simulink model "Simulation"  (R2018a)
settings: Solver=VariableStepAuto  StartTime=0.0  StopTime=10  FixedStep=1e-6  MaxStep=Tsc  RelTol=1e-3  EnableMultiTasking=on
InitFcn:
  | clc
  | close all
  | clear all
  | 
  | %Vector-space-decomposition transform (2)
  | D = 2/6*[cos(0) cos(1*pi/3) cos(2*pi/3) cos(3*pi/3) cos(4*pi/3) cos(5*pi/3);
  |         sin(0) sin(1*pi/3) sin(2*pi/3) sin(3*pi/3) sin(4*pi/3) sin(5*pi/3);
  |         cos(2*0) cos(2*pi/3) cos(4*pi/3) cos(6*pi/3) cos(8*pi/3) cos(10*pi/3);
  |         sin(2*0) sin(2*pi/3) sin(4*pi/3) sin(6*pi/3) sin(8*pi/3) sin(10*pi/3);
  |         1/2 1/2  1/2 1/2 1/2 1/2;
  |         1/2 -1/2 1/2 -1/2 1/2 -1/2];
  | 
  | %Control sampling period
  | Tsc = 1e-4;
  | 
  | %Parameters of six-phase induction machine (other than stator resistance):
  | P=2; %Number of machine pole pairs
  | Lm=284e-3; %alpha-beta magnetizing inductance (mH)
  | Rr=2.9; %alpha-beta rotor resistance (ohm)
  | Lls=10e-3; %alpha-beta stator leakage inductance (mH)
  | Llr=21e-3; %alpha-beta rotor leakage inductance (mH)
  | Lxy=4.52e-3; %xy stator inductance (mH)
  | L0=24.5e-3; %0- stator inductance (mH)
  | J=0.0261; %Inertia (Kg*m^2)
  | f=0.0033; %Friction coefficient (N*m*s)
  | Ls = Lls+Lm; Lr = Llr+Lm;  %alpha-beta self-inductances (mH)
undefined symbols (not defined in the file): DiscIntNeverNeededParam
libraries: powerlib x37, simulink x20, simulink_extras x7
(part 2 of 3)

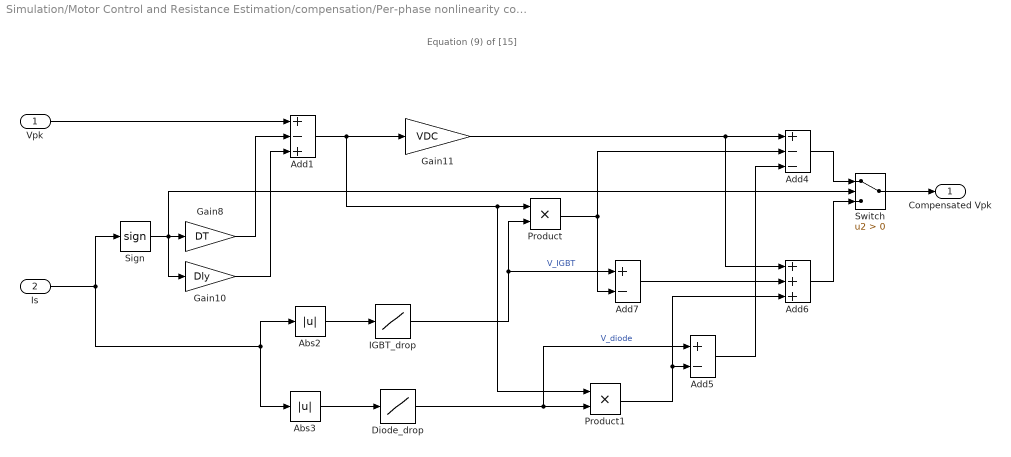
== system Simulation/Motor Control and Resistance Estimation/compensation/Per-phase nonlinearity comp. a ==
  note: Equation (9) of [15]
  Vpk : Inport
  Is : Inport  Port=2
  Abs2 : Abs
  Abs3 : Abs
  Add1 : Sum  Inputs=+-+
  Add4 : Sum  Inputs=+--
  Add5 : Sum  Inputs=+-
  Add6 : Sum  Inputs=+++
  Add7 : Sum  Inputs=+-
  Diode_drop : Lookup_n-D  NumberOfTableDimensions=1  BreakpointsForDimension1=|  Table=|  InternalRulePriority=Speed  RndMeth=Simplest  InputSameDT=on
      BreakpointsForDimension1=|
      | [0
      | 0.133928966
      | 0.255064642
      | 0.474221552
      | 0.729904408
      | 0.949060092
      | 1.31432079
      | 1.606529594
      | 1.935264345
      | 2.337050991
      | 2.665784516
      | 3.031045214
      | 3.286728071
      | 3.688514717
      | 4.090301362
      | 4.528613955
      | 4.966926548
      | 5.369012486
      | 6.011863029
      | 6.494000937
      | 6.895782526
      | 7.538633069
      | 7.940414658
      | 8.392857318
      | 9.017857931
      | 9.508928352
      | 10.04464299
      | 10.53571464
      | 11.07142805
      | 11.60714268
      | 12.09821433
      | ]
      Table=|
      | [0.649155738
      | 0.724202664
      | 0.757646637
      | 0.789882494
      | 0.820583364
      | 0.852819221
      | 0.883520091
      | 0.906545718
      | 0.924966281
      | 0.949526998
      | 0.971017535
      | 0.987903009
      | 1.006323572
      | 1.021673955
      | 1.040094519
      | 1.058514979
      | 1.075400452
      | 1.095506677
      | 1.110703514
      | 1.130965963
      | 1.15291695
      | 1.164736713
      | 1.184999162
      | 1.206378996
      | 1.217636169
      | 1.228893136
      | 1.240150103
      | 1.255159529
      | 1.264540369
      | 1.281425922
      | 1.300187602
      | ]
  Gain10 : Gain  Gain=Dly
  Gain11 : Gain  Gain=VDC
  Gain8 : Gain  Gain=DT
  IGBT_drop : Lookup_n-D  NumberOfTableDimensions=1  BreakpointsForDimension1=|  Table=|  InternalRulePriority=Speed  RndMeth=Simplest  InputSameDT=on
      BreakpointsForDimension1=|
      | [0
      | 0.18153084
      | 0.386589315
      | 0.625825349
      | 0.933414208
      | 1.309355891
      | 1.651121163
      | 2.129592084
      | 2.53971018
      | 3.052357513
      | 3.530829581
      | 3.872593705
      | 4.385242186
      | 4.658654632
      | 5.034596316
      | 5.37636044
      | 5.752302124
      | 6.059890983
      | 6.401656254
      | 6.743421525
      | 7.085186797
      | 7.426952068
      | 7.802893752
      | 8.110482611
      | 8.38389391
      | 8.588953532
      | 8.89654239
      | 9.238307662
      | 9.443366136
      | 9.68260217
      | 9.921837631
      | 10.22942592
      | 10.53701477
      | 10.91295646
      | 11.11801551
      | 11.39142738
      | 11.73319265
      | 12.04078151
      | ]
      Table=|
      | [0.58448405
      | 0.632969591
      | 0.671758056
      | 0.708122171
      | 0.739637748
      | 0.783274751
      | 0.817214515
      | 0.858427331
      | 0.880245832
      | 0.899639983
      | 0.921458485
      | 0.948125524
      | 0.969944025
      | 0.984489639
      | 1.00388379
      | 1.023278104
      | 1.037823717
      | 1.059642218
      | 1.071763644
      | 1.086309258
      | 1.100854871
      | 1.112976297
      | 1.12752191
      | 1.144491874
      | 1.154188949
      | 1.166310375
      | 1.173583101
      | 1.188128877
      | 1.197825952
      | 1.209947378
      | 1.222068641
      | 1.234190067
      | 1.239038605
      | 1.246311493
      | 1.258432919
      | 1.270554182
      | 1.280251257
      | 1.289948496
      | ]
  Product : Product
  Product1 : Product
  Sign : Signum
  Switch : Switch  Criteria=u2 > Threshold
  Compensated Vpk : Outport
  wires:
  Add6/1 -> Switch/3
  Is/1 -> Abs3/1, Abs2/1, Sign/1
  Product1/1 -> Add6/3, Add5/2
  Add1/1 -> Product1/1, Product/1, Gain11/1
  Product/1 -> Add7/2, Add4/2
  Diode_drop/1 -> Add5/1, Product1/2  "V_diode"
  Sign/1 -> Switch/2, Gain10/1, Gain8/1
  Add7/1 -> Add6/2
  Gain11/1 -> Add6/1, Add4/1
  Add4/1 -> Switch/1
  Gain8/1 -> Add1/2
  IGBT_drop/1 -> Add7/1, Product/2  "V_IGBT"
  Add5/1 -> Add4/3
  Abs2/1 -> IGBT_drop/1
  Gain10/1 -> Add1/3
  Switch/1 -> Compensated Vpk/1
  Vpk/1 -> Add1/1
  Abs3/1 -> Diode_drop/1

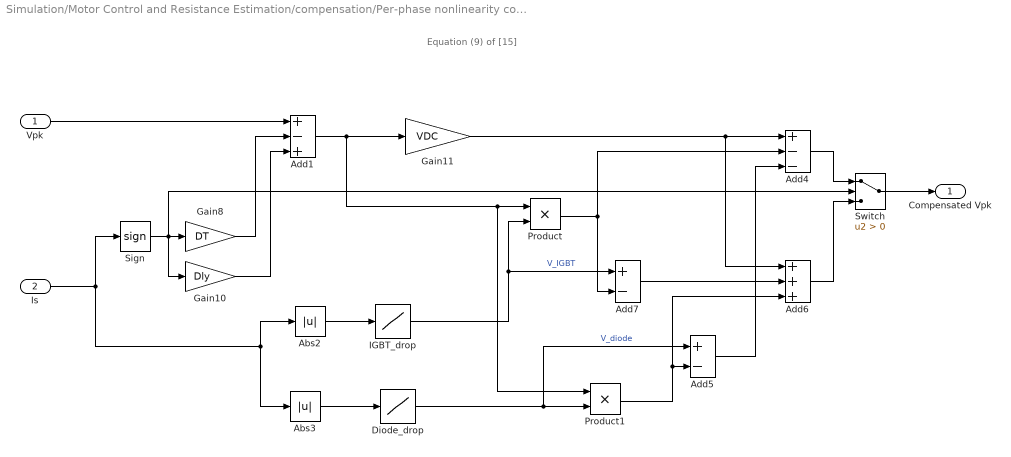
== system Simulation/Motor Control and Resistance Estimation/compensation/Per-phase nonlinearity comp. b ==
  note: Equation (9) of [15]
  Vpk : Inport
  Is : Inport  Port=2
  Abs2 : Abs
  Abs3 : Abs
  Add1 : Sum  Inputs=+-+
  Add4 : Sum  Inputs=+--
  Add5 : Sum  Inputs=+-
  Add6 : Sum  Inputs=+++
  Add7 : Sum  Inputs=+-
  Diode_drop : Lookup_n-D  NumberOfTableDimensions=1  BreakpointsForDimension1=|  Table=|  InternalRulePriority=Speed  RndMeth=Simplest  InputSameDT=on
      BreakpointsForDimension1=|
      | [0
      | 0.133928966
      | 0.255064642
      | 0.474221552
      | 0.729904408
      | 0.949060092
      | 1.31432079
      | 1.606529594
      | 1.935264345
      | 2.337050991
      | 2.665784516
      | 3.031045214
      | 3.286728071
      | 3.688514717
      | 4.090301362
      | 4.528613955
      | 4.966926548
      | 5.369012486
      | 6.011863029
      | 6.494000937
      | 6.895782526
      | 7.538633069
      | 7.940414658
      | 8.392857318
      | 9.017857931
      | 9.508928352
      | 10.04464299
      | 10.53571464
      | 11.07142805
      | 11.60714268
      | 12.09821433
      | ]
      Table=|
      | [0.649155738
      | 0.724202664
      | 0.757646637
      | 0.789882494
      | 0.820583364
      | 0.852819221
      | 0.883520091
      | 0.906545718
      | 0.924966281
      | 0.949526998
      | 0.971017535
      | 0.987903009
      | 1.006323572
      | 1.021673955
      | 1.040094519
      | 1.058514979
      | 1.075400452
      | 1.095506677
      | 1.110703514
      | 1.130965963
      | 1.15291695
      | 1.164736713
      | 1.184999162
      | 1.206378996
      | 1.217636169
      | 1.228893136
      | 1.240150103
      | 1.255159529
      | 1.264540369
      | 1.281425922
      | 1.300187602
      | ]
  Gain10 : Gain  Gain=Dly
  Gain11 : Gain  Gain=VDC
  Gain8 : Gain  Gain=DT
  IGBT_drop : Lookup_n-D  NumberOfTableDimensions=1  BreakpointsForDimension1=|  Table=|  InternalRulePriority=Speed  RndMeth=Simplest  InputSameDT=on
      BreakpointsForDimension1=|
      | [0
      | 0.18153084
      | 0.386589315
      | 0.625825349
      | 0.933414208
      | 1.309355891
      | 1.651121163
      | 2.129592084
      | 2.53971018
      | 3.052357513
      | 3.530829581
      | 3.872593705
      | 4.385242186
      | 4.658654632
      | 5.034596316
      | 5.37636044
      | 5.752302124
      | 6.059890983
      | 6.401656254
      | 6.743421525
      | 7.085186797
      | 7.426952068
      | 7.802893752
      | 8.110482611
      | 8.38389391
      | 8.588953532
      | 8.89654239
      | 9.238307662
      | 9.443366136
      | 9.68260217
      | 9.921837631
      | 10.22942592
      | 10.53701477
      | 10.91295646
      | 11.11801551
      | 11.39142738
      | 11.73319265
      | 12.04078151
      | ]
      Table=|
      | [0.58448405
      | 0.632969591
      | 0.671758056
      | 0.708122171
      | 0.739637748
      | 0.783274751
      | 0.817214515
      | 0.858427331
      | 0.880245832
      | 0.899639983
      | 0.921458485
      | 0.948125524
      | 0.969944025
      | 0.984489639
      | 1.00388379
      | 1.023278104
      | 1.037823717
      | 1.059642218
      | 1.071763644
      | 1.086309258
      | 1.100854871
      | 1.112976297
      | 1.12752191
      | 1.144491874
      | 1.154188949
      | 1.166310375
      | 1.173583101
      | 1.188128877
      | 1.197825952
      | 1.209947378
      | 1.222068641
      | 1.234190067
      | 1.239038605
      | 1.246311493
      | 1.258432919
      | 1.270554182
      | 1.280251257
      | 1.289948496
      | ]
  Product : Product
  Product1 : Product
  Sign : Signum
  Switch : Switch  Criteria=u2 > Threshold
  Compensated Vpk : Outport
  wires:
  Abs3/1 -> Diode_drop/1
  Vpk/1 -> Add1/1
  Switch/1 -> Compensated Vpk/1
  Gain10/1 -> Add1/3
  Abs2/1 -> IGBT_drop/1
  Add5/1 -> Add4/3
  IGBT_drop/1 -> Product/2, Add7/1  "V_IGBT"
  Gain8/1 -> Add1/2
  Add4/1 -> Switch/1
  Gain11/1 -> Add4/1, Add6/1
  Add7/1 -> Add6/2
  Sign/1 -> Gain8/1, Gain10/1, Switch/2
  Diode_drop/1 -> Product1/2, Add5/1  "V_diode"
  Product/1 -> Add4/2, Add7/2
  Add1/1 -> Gain11/1, Product/1, Product1/1
  Product1/1 -> Add5/2, Add6/3
  Is/1 -> Sign/1, Abs2/1, Abs3/1
  Add6/1 -> Switch/3

== system Simulation/Motor Control and Resistance Estimation/compensation/Per-phase nonlinearity comp. c ==
  note: Equation (9) of [15]
  Vpk : Inport
  Is : Inport  Port=2
  Abs2 : Abs
  Abs3 : Abs
  Add1 : Sum  Inputs=+-+
  Add4 : Sum  Inputs=+--
  Add5 : Sum  Inputs=+-
  Add6 : Sum  Inputs=+++
  Add7 : Sum  Inputs=+-
  Diode_drop : Lookup_n-D  NumberOfTableDimensions=1  BreakpointsForDimension1=|  Table=|  InternalRulePriority=Speed  RndMeth=Simplest  InputSameDT=on
      BreakpointsForDimension1=|
      | [0
      | 0.133928966
      | 0.255064642
      | 0.474221552
      | 0.729904408
      | 0.949060092
      | 1.31432079
      | 1.606529594
      | 1.935264345
      | 2.337050991
      | 2.665784516
      | 3.031045214
      | 3.286728071
      | 3.688514717
      | 4.090301362
      | 4.528613955
      | 4.966926548
      | 5.369012486
      | 6.011863029
      | 6.494000937
      | 6.895782526
      | 7.538633069
      | 7.940414658
      | 8.392857318
      | 9.017857931
      | 9.508928352
      | 10.04464299
      | 10.53571464
      | 11.07142805
      | 11.60714268
      | 12.09821433
      | ]
      Table=|
      | [0.649155738
      | 0.724202664
      | 0.757646637
      | 0.789882494
      | 0.820583364
      | 0.852819221
      | 0.883520091
      | 0.906545718
      | 0.924966281
      | 0.949526998
      | 0.971017535
      | 0.987903009
      | 1.006323572
      | 1.021673955
      | 1.040094519
      | 1.058514979
      | 1.075400452
      | 1.095506677
      | 1.110703514
      | 1.130965963
      | 1.15291695
      | 1.164736713
      | 1.184999162
      | 1.206378996
      | 1.217636169
      | 1.228893136
      | 1.240150103
      | 1.255159529
      | 1.264540369
      | 1.281425922
      | 1.300187602
      | ]
  Gain10 : Gain  Gain=Dly
  Gain11 : Gain  Gain=VDC
  Gain8 : Gain  Gain=DT
  IGBT_drop : Lookup_n-D  NumberOfTableDimensions=1  BreakpointsForDimension1=|  Table=|  InternalRulePriority=Speed  RndMeth=Simplest  InputSameDT=on
      BreakpointsForDimension1=|
      | [0
      | 0.18153084
      | 0.386589315
      | 0.625825349
      | 0.933414208
      | 1.309355891
      | 1.651121163
      | 2.129592084
      | 2.53971018
      | 3.052357513
      | 3.530829581
      | 3.872593705
      | 4.385242186
      | 4.658654632
      | 5.034596316
      | 5.37636044
      | 5.752302124
      | 6.059890983
      | 6.401656254
      | 6.743421525
      | 7.085186797
      | 7.426952068
      | 7.802893752
      | 8.110482611
      | 8.38389391
      | 8.588953532
      | 8.89654239
      | 9.238307662
      | 9.443366136
      | 9.68260217
      | 9.921837631
      | 10.22942592
      | 10.53701477
      | 10.91295646
      | 11.11801551
      | 11.39142738
      | 11.73319265
      | 12.04078151
      | ]
      Table=|
      | [0.58448405
      | 0.632969591
      | 0.671758056
      | 0.708122171
      | 0.739637748
      | 0.783274751
      | 0.817214515
      | 0.858427331
      | 0.880245832
      | 0.899639983
      | 0.921458485
      | 0.948125524
      | 0.969944025
      | 0.984489639
      | 1.00388379
      | 1.023278104
      | 1.037823717
      | 1.059642218
      | 1.071763644
      | 1.086309258
      | 1.100854871
      | 1.112976297
      | 1.12752191
      | 1.144491874
      | 1.154188949
      | 1.166310375
      | 1.173583101
      | 1.188128877
      | 1.197825952
      | 1.209947378
      | 1.222068641
      | 1.234190067
      | 1.239038605
      | 1.246311493
      | 1.258432919
      | 1.270554182
      | 1.280251257
      | 1.289948496
      | ]
  Product : Product
  Product1 : Product
  Sign : Signum
  Switch : Switch  Criteria=u2 > Threshold
  Compensated Vpk : Outport
  wires:
  Add6/1 -> Switch/3
  Is/1 -> Abs3/1, Abs2/1, Sign/1
  Product1/1 -> Add6/3, Add5/2
  Add1/1 -> Product1/1, Product/1, Gain11/1
  Product/1 -> Add7/2, Add4/2
  Diode_drop/1 -> Add5/1, Product1/2  "V_diode"
  Sign/1 -> Switch/2, Gain10/1, Gain8/1
  Add7/1 -> Add6/2
  Gain11/1 -> Add6/1, Add4/1
  Add4/1 -> Switch/1
  Gain8/1 -> Add1/2
  IGBT_drop/1 -> Add7/1, Product/2  "V_IGBT"
  Add5/1 -> Add4/3
  Abs2/1 -> IGBT_drop/1
  Gain10/1 -> Add1/3
  Switch/1 -> Compensated Vpk/1
  Vpk/1 -> Add1/1
  Abs3/1 -> Diode_drop/1

== system Simulation/Motor Control and Resistance Estimation/compensation/Per-phase nonlinearity comp. d ==
  note: Equation (9) of [15]
  Vpk : Inport
  Is : Inport  Port=2
  Abs2 : Abs
  Abs3 : Abs
  Add1 : Sum  Inputs=+-+
  Add4 : Sum  Inputs=+--
  Add5 : Sum  Inputs=+-
  Add6 : Sum  Inputs=+++
  Add7 : Sum  Inputs=+-
  Diode_drop : Lookup_n-D  NumberOfTableDimensions=1  BreakpointsForDimension1=|  Table=|  InternalRulePriority=Speed  RndMeth=Simplest  InputSameDT=on
      BreakpointsForDimension1=|
      | [0
      | 0.133928966
      | 0.255064642
      | 0.474221552
      | 0.729904408
      | 0.949060092
      | 1.31432079
      | 1.606529594
      | 1.935264345
      | 2.337050991
      | 2.665784516
      | 3.031045214
      | 3.286728071
      | 3.688514717
      | 4.090301362
      | 4.528613955
      | 4.966926548
      | 5.369012486
      | 6.011863029
      | 6.494000937
      | 6.895782526
      | 7.538633069
      | 7.940414658
      | 8.392857318
      | 9.017857931
      | 9.508928352
      | 10.04464299
      | 10.53571464
      | 11.07142805
      | 11.60714268
      | 12.09821433
      | ]
      Table=|
      | [0.649155738
      | 0.724202664
      | 0.757646637
      | 0.789882494
      | 0.820583364
      | 0.852819221
      | 0.883520091
      | 0.906545718
      | 0.924966281
      | 0.949526998
      | 0.971017535
      | 0.987903009
      | 1.006323572
      | 1.021673955
      | 1.040094519
      | 1.058514979
      | 1.075400452
      | 1.095506677
      | 1.110703514
      | 1.130965963
      | 1.15291695
      | 1.164736713
      | 1.184999162
      | 1.206378996
      | 1.217636169
      | 1.228893136
      | 1.240150103
      | 1.255159529
      | 1.264540369
      | 1.281425922
      | 1.300187602
      | ]
  Gain10 : Gain  Gain=Dly
  Gain11 : Gain  Gain=VDC
  Gain8 : Gain  Gain=DT
  IGBT_drop : Lookup_n-D  NumberOfTableDimensions=1  BreakpointsForDimension1=|  Table=|  InternalRulePriority=Speed  RndMeth=Simplest  InputSameDT=on
      BreakpointsForDimension1=|
      | [0
      | 0.18153084
      | 0.386589315
      | 0.625825349
      | 0.933414208
      | 1.309355891
      | 1.651121163
      | 2.129592084
      | 2.53971018
      | 3.052357513
      | 3.530829581
      | 3.872593705
      | 4.385242186
      | 4.658654632
      | 5.034596316
      | 5.37636044
      | 5.752302124
      | 6.059890983
      | 6.401656254
      | 6.743421525
      | 7.085186797
      | 7.426952068
      | 7.802893752
      | 8.110482611
      | 8.38389391
      | 8.588953532
      | 8.89654239
      | 9.238307662
      | 9.443366136
      | 9.68260217
      | 9.921837631
      | 10.22942592
      | 10.53701477
      | 10.91295646
      | 11.11801551
      | 11.39142738
      | 11.73319265
      | 12.04078151
      | ]
      Table=|
      | [0.58448405
      | 0.632969591
      | 0.671758056
      | 0.708122171
      | 0.739637748
      | 0.783274751
      | 0.817214515
      | 0.858427331
      | 0.880245832
      | 0.899639983
      | 0.921458485
      | 0.948125524
      | 0.969944025
      | 0.984489639
      | 1.00388379
      | 1.023278104
      | 1.037823717
      | 1.059642218
      | 1.071763644
      | 1.086309258
      | 1.100854871
      | 1.112976297
      | 1.12752191
      | 1.144491874
      | 1.154188949
      | 1.166310375
      | 1.173583101
      | 1.188128877
      | 1.197825952
      | 1.209947378
      | 1.222068641
      | 1.234190067
      | 1.239038605
      | 1.246311493
      | 1.258432919
      | 1.270554182
      | 1.280251257
      | 1.289948496
      | ]
  Product : Product
  Product1 : Product
  Sign : Signum
  Switch : Switch  Criteria=u2 > Threshold
  Compensated Vpk : Outport
  wires:
  Abs3/1 -> Diode_drop/1
  Vpk/1 -> Add1/1
  Switch/1 -> Compensated Vpk/1
  Gain10/1 -> Add1/3
  Abs2/1 -> IGBT_drop/1
  Add5/1 -> Add4/3
  IGBT_drop/1 -> Product/2, Add7/1  "V_IGBT"
  Gain8/1 -> Add1/2
  Add4/1 -> Switch/1
  Gain11/1 -> Add4/1, Add6/1
  Add7/1 -> Add6/2
  Sign/1 -> Gain8/1, Gain10/1, Switch/2
  Diode_drop/1 -> Product1/2, Add5/1  "V_diode"
  Product/1 -> Add4/2, Add7/2
  Add1/1 -> Gain11/1, Product/1, Product1/1
  Product1/1 -> Add5/2, Add6/3
  Is/1 -> Sign/1, Abs2/1, Abs3/1
  Add6/1 -> Switch/3

== system Simulation/Motor Control and Resistance Estimation/compensation/Per-phase nonlinearity comp. e ==
  note: Equation (9) of [15]
  Vpk : Inport
  Is : Inport  Port=2
  Abs2 : Abs
  Abs3 : Abs
  Add1 : Sum  Inputs=+-+
  Add4 : Sum  Inputs=+--
  Add5 : Sum  Inputs=+-
  Add6 : Sum  Inputs=+++
  Add7 : Sum  Inputs=+-
  Diode_drop : Lookup_n-D  NumberOfTableDimensions=1  BreakpointsForDimension1=|  Table=|  InternalRulePriority=Speed  RndMeth=Simplest  InputSameDT=on
      BreakpointsForDimension1=|
      | [0
      | 0.133928966
      | 0.255064642
      | 0.474221552
      | 0.729904408
      | 0.949060092
      | 1.31432079
      | 1.606529594
      | 1.935264345
      | 2.337050991
      | 2.665784516
      | 3.031045214
      | 3.286728071
      | 3.688514717
      | 4.090301362
      | 4.528613955
      | 4.966926548
      | 5.369012486
      | 6.011863029
      | 6.494000937
      | 6.895782526
      | 7.538633069
      | 7.940414658
      | 8.392857318
      | 9.017857931
      | 9.508928352
      | 10.04464299
      | 10.53571464
      | 11.07142805
      | 11.60714268
      | 12.09821433
      | ]
      Table=|
      | [0.649155738
      | 0.724202664
      | 0.757646637
      | 0.789882494
      | 0.820583364
      | 0.852819221
      | 0.883520091
      | 0.906545718
      | 0.924966281
      | 0.949526998
      | 0.971017535
      | 0.987903009
      | 1.006323572
      | 1.021673955
      | 1.040094519
      | 1.058514979
      | 1.075400452
      | 1.095506677
      | 1.110703514
      | 1.130965963
      | 1.15291695
      | 1.164736713
      | 1.184999162
      | 1.206378996
      | 1.217636169
      | 1.228893136
      | 1.240150103
      | 1.255159529
      | 1.264540369
      | 1.281425922
      | 1.300187602
      | ]
  Gain10 : Gain  Gain=Dly
  Gain11 : Gain  Gain=VDC
  Gain8 : Gain  Gain=DT
  IGBT_drop : Lookup_n-D  NumberOfTableDimensions=1  BreakpointsForDimension1=|  Table=|  InternalRulePriority=Speed  RndMeth=Simplest  InputSameDT=on
      BreakpointsForDimension1=|
      | [0
      | 0.18153084
      | 0.386589315
      | 0.625825349
      | 0.933414208
      | 1.309355891
      | 1.651121163
      | 2.129592084
      | 2.53971018
      | 3.052357513
      | 3.530829581
      | 3.872593705
      | 4.385242186
      | 4.658654632
      | 5.034596316
      | 5.37636044
      | 5.752302124
      | 6.059890983
      | 6.401656254
      | 6.743421525
      | 7.085186797
      | 7.426952068
      | 7.802893752
      | 8.110482611
      | 8.38389391
      | 8.588953532
      | 8.89654239
      | 9.238307662
      | 9.443366136
      | 9.68260217
      | 9.921837631
      | 10.22942592
      | 10.53701477
      | 10.91295646
      | 11.11801551
      | 11.39142738
      | 11.73319265
      | 12.04078151
      | ]
      Table=|
      | [0.58448405
      | 0.632969591
      | 0.671758056
      | 0.708122171
      | 0.739637748
      | 0.783274751
      | 0.817214515
      | 0.858427331
      | 0.880245832
      | 0.899639983
      | 0.921458485
      | 0.948125524
      | 0.969944025
      | 0.984489639
      | 1.00388379
      | 1.023278104
      | 1.037823717
      | 1.059642218
      | 1.071763644
      | 1.086309258
      | 1.100854871
      | 1.112976297
      | 1.12752191
      | 1.144491874
      | 1.154188949
      | 1.166310375
      | 1.173583101
      | 1.188128877
      | 1.197825952
      | 1.209947378
      | 1.222068641
      | 1.234190067
      | 1.239038605
      | 1.246311493
      | 1.258432919
      | 1.270554182
      | 1.280251257
      | 1.289948496
      | ]
  Product : Product
  Product1 : Product
  Sign : Signum
  Switch : Switch  Criteria=u2 > Threshold
  Compensated Vpk : Outport
  wires:
  Add6/1 -> Switch/3
  Is/1 -> Abs3/1, Abs2/1, Sign/1
  Product1/1 -> Add6/3, Add5/2
  Add1/1 -> Product1/1, Product/1, Gain11/1
  Product/1 -> Add7/2, Add4/2
  Diode_drop/1 -> Add5/1, Product1/2  "V_diode"
  Sign/1 -> Switch/2, Gain10/1, Gain8/1
  Add7/1 -> Add6/2
  Gain11/1 -> Add6/1, Add4/1
  Add4/1 -> Switch/1
  Gain8/1 -> Add1/2
  IGBT_drop/1 -> Add7/1, Product/2  "V_IGBT"
  Add5/1 -> Add4/3
  Abs2/1 -> IGBT_drop/1
  Gain10/1 -> Add1/3
  Switch/1 -> Compensated Vpk/1
  Vpk/1 -> Add1/1
  Abs3/1 -> Diode_drop/1

== system Simulation/Motor Control and Resistance Estimation/compensation/Per-phase nonlinearity comp. f ==
  note: Equation (9) of [15]
  Vpk : Inport
  Is : Inport  Port=2
  Abs2 : Abs
  Abs3 : Abs
  Add1 : Sum  Inputs=+-+
  Add4 : Sum  Inputs=+--
  Add5 : Sum  Inputs=+-
  Add6 : Sum  Inputs=+++
  Add7 : Sum  Inputs=+-
  Diode_drop : Lookup_n-D  NumberOfTableDimensions=1  BreakpointsForDimension1=|  Table=|  InternalRulePriority=Speed  RndMeth=Simplest  InputSameDT=on
      BreakpointsForDimension1=|
      | [0
      | 0.133928966
      | 0.255064642
      | 0.474221552
      | 0.729904408
      | 0.949060092
      | 1.31432079
      | 1.606529594
      | 1.935264345
      | 2.337050991
      | 2.665784516
      | 3.031045214
      | 3.286728071
      | 3.688514717
      | 4.090301362
      | 4.528613955
      | 4.966926548
      | 5.369012486
      | 6.011863029
      | 6.494000937
      | 6.895782526
      | 7.538633069
      | 7.940414658
      | 8.392857318
      | 9.017857931
      | 9.508928352
      | 10.04464299
      | 10.53571464
      | 11.07142805
      | 11.60714268
      | 12.09821433
      | ]
      Table=|
      | [0.649155738
      | 0.724202664
      | 0.757646637
      | 0.789882494
      | 0.820583364
      | 0.852819221
      | 0.883520091
      | 0.906545718
      | 0.924966281
      | 0.949526998
      | 0.971017535
      | 0.987903009
      | 1.006323572
      | 1.021673955
      | 1.040094519
      | 1.058514979
      | 1.075400452
      | 1.095506677
      | 1.110703514
      | 1.130965963
      | 1.15291695
      | 1.164736713
      | 1.184999162
      | 1.206378996
      | 1.217636169
      | 1.228893136
      | 1.240150103
      | 1.255159529
      | 1.264540369
      | 1.281425922
      | 1.300187602
      | ]
  Gain10 : Gain  Gain=Dly
  Gain11 : Gain  Gain=VDC
  Gain8 : Gain  Gain=DT
  IGBT_drop : Lookup_n-D  NumberOfTableDimensions=1  BreakpointsForDimension1=|  Table=|  InternalRulePriority=Speed  RndMeth=Simplest  InputSameDT=on
      BreakpointsForDimension1=|
      | [0
      | 0.18153084
      | 0.386589315
      | 0.625825349
      | 0.933414208
      | 1.309355891
      | 1.651121163
      | 2.129592084
      | 2.53971018
      | 3.052357513
      | 3.530829581
      | 3.872593705
      | 4.385242186
      | 4.658654632
      | 5.034596316
      | 5.37636044
      | 5.752302124
      | 6.059890983
      | 6.401656254
      | 6.743421525
      | 7.085186797
      | 7.426952068
      | 7.802893752
      | 8.110482611
      | 8.38389391
      | 8.588953532
      | 8.89654239
      | 9.238307662
      | 9.443366136
      | 9.68260217
      | 9.921837631
      | 10.22942592
      | 10.53701477
      | 10.91295646
      | 11.11801551
      | 11.39142738
      | 11.73319265
      | 12.04078151
      | ]
      Table=|
      | [0.58448405
      | 0.632969591
      | 0.671758056
      | 0.708122171
      | 0.739637748
      | 0.783274751
      | 0.817214515
      | 0.858427331
      | 0.880245832
      | 0.899639983
      | 0.921458485
      | 0.948125524
      | 0.969944025
      | 0.984489639
      | 1.00388379
      | 1.023278104
      | 1.037823717
      | 1.059642218
      | 1.071763644
      | 1.086309258
      | 1.100854871
      | 1.112976297
      | 1.12752191
      | 1.144491874
      | 1.154188949
      | 1.166310375
      | 1.173583101
      | 1.188128877
      | 1.197825952
      | 1.209947378
      | 1.222068641
      | 1.234190067
      | 1.239038605
      | 1.246311493
      | 1.258432919
      | 1.270554182
      | 1.280251257
      | 1.289948496
      | ]
  Product : Product
  Product1 : Product
  Sign : Signum
  Switch : Switch  Criteria=u2 > Threshold
  Compensated Vpk : Outport
  wires:
  Abs3/1 -> Diode_drop/1
  Vpk/1 -> Add1/1
  Switch/1 -> Compensated Vpk/1
  Gain10/1 -> Add1/3
  Abs2/1 -> IGBT_drop/1
  Add5/1 -> Add4/3
  IGBT_drop/1 -> Product/2, Add7/1  "V_IGBT"
  Gain8/1 -> Add1/2
  Add4/1 -> Switch/1
  Gain11/1 -> Add4/1, Add6/1
  Add7/1 -> Add6/2
  Sign/1 -> Gain8/1, Gain10/1, Switch/2
  Diode_drop/1 -> Product1/2, Add5/1  "V_diode"
  Product/1 -> Add4/2, Add7/2
  Add1/1 -> Gain11/1, Product/1, Product1/1
  Product1/1 -> Add5/2, Add6/3
  Is/1 -> Sign/1, Abs2/1, Abs3/1
  Add6/1 -> Switch/3

== system Simulation/Six-phase induction machine with extra per-phase stator resistances/Symmetrical six-phase induction machine with balanced stator resistances/0- circuit ==
  note: Lamda
  V0 : Inport
  Integrator : Integrator
  R : Gain  Gain=R0  Multiplication=Matrix(K*u)  SaturateOnIntegerOverflow=on  OutDataTypeStr=Inherit: Same as input  ParamDataTypeStr=Inherit: Same as input
  Sum : Sum  Inputs=+-  SaturateOnIntegerOverflow=on
  inv(L) : Gain  Gain=1/L0  Multiplication=Matrix(K*u)  SaturateOnIntegerOverflow=on  OutDataTypeStr=Inherit: Same as input  ParamDataTypeStr=Inherit: Same as input
  i0 : Outport  VectorParamsAs1DForOutWhenUnconnected=off
  wires:
  Sum/1 -> Integrator/1
  Integrator/1 -> inv(L)/1
  inv(L)/1 -> R/1, i0/1
  R/1 -> Sum/2
  V0/1 -> Sum/1

== system Simulation/Six-phase induction machine with extra per-phase stator resistances/Symmetrical six-phase induction machine with balanced stator resistances/Mechanical model ==
  T : Inport
  No : Inport  Port=2
  Gain : Gain  Gain=1/J
  Gain1 : Gain  Gain=f
  Integrator : Integrator  InitialConditionSource=external  InitialCondition=1000*2*pi/60
  Sum1 : Sum  Inputs=+-  InputSameDT=on  SaturateOnIntegerOverflow=on  OutDataTypeStr=Inherit: Same as first input
  rpm to rad/s : Gain  Gain=2*pi/60
  wm : Outport
  wires:
  Gain/1 -> Integrator/1
  Sum1/1 -> Gain/1
  rpm to rad/s/1 -> Integrator/2
  Integrator/1 -> wm/1, Gain1/1  "Speed (rad/s)"
  Gain1/1 -> Sum1/2
  No/1 -> rpm to rad/s/1  "Initial speed (rpm)"
  T/1 -> Sum1/1  "Electromagnetic torque (Nm)"

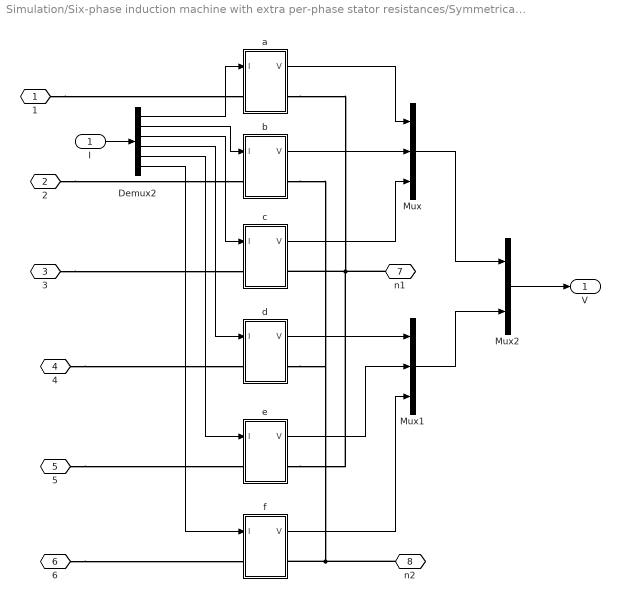
== system Simulation/Six-phase induction machine with extra per-phase stator resistances/Symmetrical six-phase induction machine with balanced stator resistances/Subsystem ==
  I : Inport
  Demux2 : Demux  Outputs=6
      settings: DisplayOption=none
  Mux : Mux  Inputs=3
  Mux1 : Mux  Inputs=3
  Mux2 : Mux  Inputs=2
  a : Subsystem
  b : Subsystem
  c : Subsystem
  d : Subsystem
  e : Subsystem
  f : Subsystem
  1 : PMIOPort  Side=Left
  2 : PMIOPort  Port=2  Side=Left
  3 : PMIOPort  Port=3  Side=Left
  4 : PMIOPort  Port=4  Side=Left
  5 : PMIOPort  Port=5  Side=Left
  6 : PMIOPort  Port=6  Side=Left
  n1 : PMIOPort  Port=7  Side=Right
  n2 : PMIOPort  Port=8  Side=Right
  V : Outport  VectorParamsAs1DForOutWhenUnconnected=off
  wires:
  I/1 -> Demux2/1
  Demux2/1 -> a/1(I)
  Demux2/2 -> b/1(I)
  Demux2/3 -> c/1(I)
  Demux2/4 -> d/1(I)
  Demux2/5 -> e/1(I)
  Demux2/6 -> f/1(I)
  b/1(V) -> Mux/2
  c/1(V) -> Mux/3
  a/1(V) -> Mux/1
  d/1(V) -> Mux1/1
  e/1(V) -> Mux1/2
  f/1(V) -> Mux1/3
  Mux/1 -> Mux2/1
  Mux1/1 -> Mux2/2
  Mux2/1 -> V/1
  connections:
  3/RConn1 -- c/LConn1
  2/RConn1 -- b/LConn1
  1/RConn1 -- a/LConn1
  n2/RConn1 -- d/RConn1 -- b/RConn1 -- f/RConn1
  4/RConn1 -- d/LConn1
  5/RConn1 -- e/LConn1
  6/RConn1 -- f/LConn1
  n1/RConn1 -- e/RConn1 -- a/RConn1 -- c/RConn1

== system Simulation/Six-phase induction machine with extra per-phase stator resistances/Symmetrical six-phase induction machine with balanced stator resistances/alpha-beta circuit ==
  note: Lamda
  Vab : Inport
  wr : Inport  Port=2
  G : Gain  Gain=G1  Multiplication=Matrix(K*u)  SaturateOnIntegerOverflow=on  OutDataTypeStr=Inherit: Same as input  ParamDataTypeStr=Inherit: Same as input
  Integrator : Integrator
  Mux1 : Mux  Inputs=2
  Pole pairs : Gain  Gain=P  SaturateOnIntegerOverflow=on  OutDataTypeStr=Inherit: Same as input  ParamDataTypeStr=Inherit: Same as input
  Product : Product  SaturateOnIntegerOverflow=on  OutDataTypeStr=Inherit: Same as first input
  R : Gain  Gain=R1  Multiplication=Matrix(K*u)  SaturateOnIntegerOverflow=on  OutDataTypeStr=Inherit: Same as input  ParamDataTypeStr=Inherit: Same as input
  Rotor voltage : Constant  Value=[0 0]
  Sum : Sum  Inputs=+--  SaturateOnIntegerOverflow=on
  T calculation : Fcn  Expr=3*P*Lm*(u(2)*u(3)-u(1)*u(4))
  inv(L) : Gain  Gain=inv(L1)  Multiplication=Matrix(K*u)  SaturateOnIntegerOverflow=on  OutDataTypeStr=Inherit: Same as input  ParamDataTypeStr=Inherit: Same as input
  T : Outport  VectorParamsAs1DForOutWhenUnconnected=off
  Iab : Outport  Port=2  VectorParamsAs1DForOutWhenUnconnected=off
  wires:
  Sum/1 -> Integrator/1
  Integrator/1 -> inv(L)/1, Product/1
  inv(L)/1 -> T calculation/1, R/1, Iab/1
  R/1 -> Sum/3
  Product/1 -> G/1
  G/1 -> Sum/2
  T calculation/1 -> T/1  "Electromagnetic torque (Nm)"
  Mux1/1 -> Sum/1
  Vab/1 -> Mux1/1
  Rotor voltage/1 -> Mux1/2
  wr/1 -> Pole pairs/1
  Pole pairs/1 -> Product/2

== system Simulation/Six-phase induction machine with extra per-phase stator resistances/Symmetrical six-phase induction machine with balanced stator resistances/xy circuit ==
  note: Lamda
  Vxy : Inport
  Integrator : Integrator
  R : Gain  Gain=Rxy  Multiplication=Matrix(K*u)  SaturateOnIntegerOverflow=on  OutDataTypeStr=Inherit: Same as input  ParamDataTypeStr=Inherit: Same as input
  Sum : Sum  Inputs=+-  SaturateOnIntegerOverflow=on
  inv(L) : Gain  Gain=1/Lxy  Multiplication=Matrix(K*u)  SaturateOnIntegerOverflow=on  OutDataTypeStr=Inherit: Same as input  ParamDataTypeStr=Inherit: Same as input
  ixy : Outport  VectorParamsAs1DForOutWhenUnconnected=off
  wires:
  Vxy/1 -> Sum/1
  R/1 -> Sum/2
  inv(L)/1 -> ixy/1, R/1
  Integrator/1 -> inv(L)/1
  Sum/1 -> Integrator/1

== system Simulation/Motor Control and Resistance Estimation/Proposed method/Generation of time sequence for injection/Detect falling edge ==
  In : Inport
  Compare To Constant2 : simulink/Logic and Bit Operations/Compare To Constant  relop=>=  const=1  OutDataTypeStr=boolean
  Compare To Constant3 : simulink/Logic and Bit Operations/Compare To Constant  relop=<  const=1  OutDataTypeStr=boolean
  Logical Operator : Logic  AllPortsSameDT=off  OutDataTypeStr=boolean
  delay : UnitDelay  SampleTime=-1
  Out : Outport
  wires:
  Logical Operator/1 -> Out/1
  In/1 -> Compare To Constant3/1, delay/1
  delay/1 -> Compare To Constant2/1
  Compare To Constant3/1 -> Logical Operator/1
  Compare To Constant2/1 -> Logical Operator/2

== system Simulation/Motor Control and Resistance Estimation/Proposed method/Generation of time sequence for injection/Detect rising edge1 ==
  In : Inport
  Compare To Constant : simulink/Logic and Bit Operations/Compare To Constant  relop=>=  const=1  OutDataTypeStr=boolean
  Compare To Constant1 : simulink/Logic and Bit Operations/Compare To Constant  relop=<  const=1  OutDataTypeStr=boolean
  Logical Operator : Logic  AllPortsSameDT=off  OutDataTypeStr=boolean
  delay : UnitDelay  SampleTime=-1
  Out : Outport
  wires:
  Logical Operator/1 -> Out/1
  In/1 -> Compare To Constant/1, delay/1
  Compare To Constant1/1 -> Logical Operator/2
  Compare To Constant/1 -> Logical Operator/1
  delay/1 -> Compare To Constant1/1

== system Simulation/Motor Control and Resistance Estimation/Proposed method/Generation of time sequence for injection/Detect rising edge2 ==
  In : Inport
  Compare To Constant : simulink/Logic and Bit Operations/Compare To Constant  relop=>=  const=1  OutDataTypeStr=boolean
  Compare To Constant1 : simulink/Logic and Bit Operations/Compare To Constant  relop=<  const=1  OutDataTypeStr=boolean
  Logical Operator : Logic  AllPortsSameDT=off  OutDataTypeStr=boolean
  delay : UnitDelay  SampleTime=-1
  Out : Outport
  wires:
  delay/1 -> Compare To Constant1/1
  Compare To Constant/1 -> Logical Operator/1
  Compare To Constant1/1 -> Logical Operator/2
  In/1 -> delay/1, Compare To Constant/1
  Logical Operator/1 -> Out/1

== system Simulation/Motor Control and Resistance Estimation/Proposed method/Generation of time sequence for injection/Time delay 1 ==
  In : Inport
  interval : Inport  Port=2
  Tsc : Inport  Port=3
  Data Type Conversion : DataTypeConversion
  Detect rising edge : Subsystem
  Relational Operator : RelationalOperator  OutDataTypeStr=boolean  RndMeth=Simplest
  S-R Flip-Flop1 : simulink_extras/Flip Flops/S-R Flip-Flop  initial_condition=0
  Unit Delay : UnitDelay  SampleTime=-1  HasFrameUpgradeWarning=on
  integrator : DiscreteIntegrator  gainval=1  ExternalReset=rising  InitialConditionSource=external  InitialCondition=Tsc  SampleTime=-1  ICPrevOutput=DiscIntNeverNeededParam  ICPrevScaledInput=DiscIntNeverNeededParam
  Out : Outport
  wires:
  In/1 -> Detect rising edge/1(In)
  Unit Delay/1 -> S-R Flip-Flop1/2, integrator/2
  integrator/1 -> Relational Operator/1
  Relational Operator/1 -> Unit Delay/1, Out/1
  S-R Flip-Flop1/1 -> Data Type Conversion/1
  Data Type Conversion/1 -> integrator/1
  Detect rising edge/1(Out) -> S-R Flip-Flop1/1
  interval/1 -> Relational Operator/2
  Tsc/1 -> integrator/3

== system Simulation/Motor Control and Resistance Estimation/Proposed method/Generation of time sequence for injection/Time delay 2 ==
  In : Inport
  interval : Inport  Port=2
  Tsc : Inport  Port=3
  Data Type Conversion : DataTypeConversion
  Detect rising edge : Subsystem
  Relational Operator : RelationalOperator  OutDataTypeStr=boolean  RndMeth=Simplest
  S-R Flip-Flop1 : simulink_extras/Flip Flops/S-R Flip-Flop  initial_condition=0
  Unit Delay : UnitDelay  SampleTime=-1  HasFrameUpgradeWarning=on
  integrator : DiscreteIntegrator  gainval=1  ExternalReset=rising  InitialConditionSource=external  InitialCondition=Tsc  SampleTime=-1  ICPrevOutput=DiscIntNeverNeededParam  ICPrevScaledInput=DiscIntNeverNeededParam
  Out : Outport
  wires:
  Tsc/1 -> integrator/3
  interval/1 -> Relational Operator/2
  Detect rising edge/1(Out) -> S-R Flip-Flop1/1
  Data Type Conversion/1 -> integrator/1
  S-R Flip-Flop1/1 -> Data Type Conversion/1
  Relational Operator/1 -> Out/1, Unit Delay/1
  integrator/1 -> Relational Operator/1
  Unit Delay/1 -> integrator/2, S-R Flip-Flop1/2
  In/1 -> Detect rising edge/1(In)

== system Simulation/Motor Control and Resistance Estimation/Proposed method/Generation of time sequence for injection/Time delay 3 ==
  In : Inport
  interval : Inport  Port=2
  Tsc : Inport  Port=3
  Data Type Conversion : DataTypeConversion
  Detect rising edge : Subsystem
  Gain : Gain  Gain=2
  Relational Operator : RelationalOperator  OutDataTypeStr=boolean  RndMeth=Simplest
  S-R Flip-Flop1 : simulink_extras/Flip Flops/S-R Flip-Flop  initial_condition=0
  Unit Delay : UnitDelay  SampleTime=-1  HasFrameUpgradeWarning=on
  integrator : DiscreteIntegrator  gainval=1  ExternalReset=rising  InitialConditionSource=external  InitialCondition=Tsc  SampleTime=-1  ICPrevOutput=DiscIntNeverNeededParam  ICPrevScaledInput=DiscIntNeverNeededParam
  Out : Outport
  wires:
  In/1 -> Detect rising edge/1(In)
  Unit Delay/1 -> S-R Flip-Flop1/2, integrator/2
  integrator/1 -> Relational Operator/1
  Relational Operator/1 -> Unit Delay/1, Out/1
  S-R Flip-Flop1/1 -> Data Type Conversion/1
  Data Type Conversion/1 -> integrator/1
  Detect rising edge/1(Out) -> S-R Flip-Flop1/1
  interval/1 -> Relational Operator/2
  Tsc/1 -> Gain/1
  Gain/1 -> integrator/3

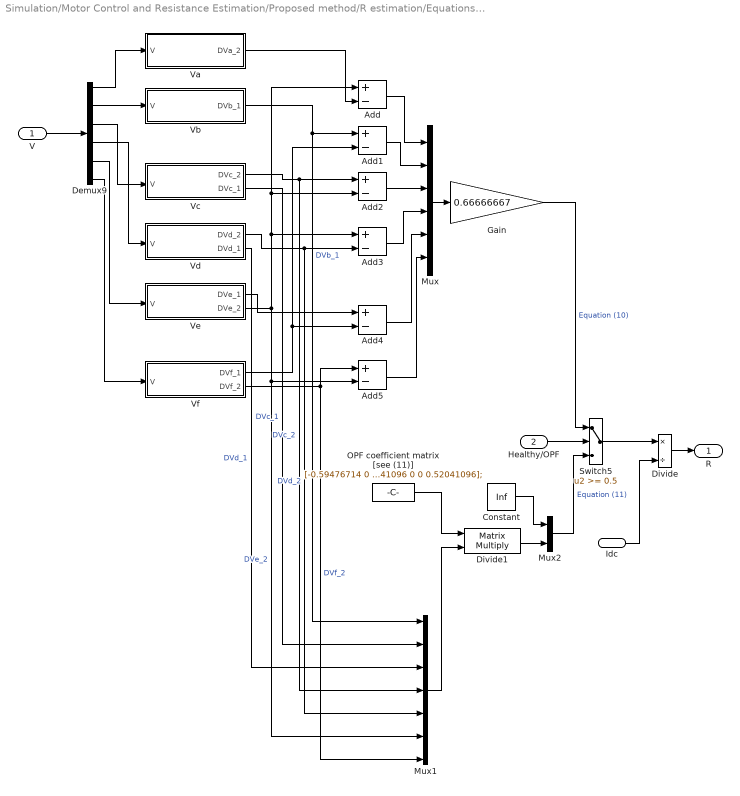
== system Simulation/Motor Control and Resistance Estimation/Proposed method/R estimation/Equations (10) & (11) ==
  V : Inport
  Healthy/OPF : Inport  Port=2
  Idc : Inport  Port=3
  Add{,1..5} (6 alike) : Sum  Inputs=+-
  Constant : Constant  Value=Inf
  Demux9 : Demux  Outputs=6
  Divide : Product  Inputs=*/
  Divide1 : Product  Inputs=**  Multiplication=Matrix(*)
  Gain : Gain  Gain=0.66666667
  Mux : Mux  Inputs=6
  Mux1 : Mux  Inputs=7
  Mux2 : Mux  Inputs=2
  OPF coefficient matrix [see (11)] : Constant  Value=|
      | [-0.59476714 0 0.59476714 0 0 0 0;
      | 0 0.59476714 -0.59476714 0 0 0 0;
      | 0 0.59460248 -0.59460248 -1.0406778 1.0406778 0 0;
      | 0 -0.23786733 0.23786733 0.41631724 0 -0.41631724 0;
      | 0 0.2973424 -0.2973424 -0.52041096 0 0 0.52041096];
  Switch5 : Switch  Threshold=0.5  SaturateOnIntegerOverflow=on
  Va : Subsystem
  Vb : Subsystem
  Vc : Subsystem
  Vd : Subsystem
  Ve : Subsystem
  Vf : Subsystem
  R : Outport
  wires:
  Vf/2(DVf_2) -> Mux1/7, Add5/1  "DVf_2"
  Vd/1(DVd_2) -> Mux1/5, Add3/2  "DVd_2"
  Mux/1 -> Gain/1
  Va/1(DVa_2) -> Add/2
  Divide/1 -> R/1
  OPF coefficient matrix [see (11)]/1 -> Divide1/1
  Vf/1(DVf_1) -> Add4/2, Add1/2
  Add4/1 -> Mux/5
  Idc/1 -> Divide/2
  Ve/2(DVe_2) -> Add5/2, Mux1/6, Add3/1, Add2/2, Add/1  "DVe_2"
  Demux9/3 -> Vc/1(V)
  Vb/1(DVb_1) -> Add1/1, Mux1/1  "DVb_1"
  Add5/1 -> Mux/6
  Demux9/6 -> Vf/1(V)
  Demux9/4 -> Vd/1(V)
  Demux9/2 -> Vb/1(V)
  Mux1/1 -> Divide1/2
  Vc/2(DVc_1) -> Mux1/2  "DVc_1"
  Add2/1 -> Mux/3
  Add1/1 -> Mux/2
  Vc/1(DVc_2) -> Mux1/4, Add2/1  "DVc_2"
  Healthy/OPF/1 -> Switch5/2
  Demux9/5 -> Ve/1(V)
  Ve/1(DVe_1) -> Add4/1
  Add/1 -> Mux/1
  Add3/1 -> Mux/4
  Switch5/1 -> Divide/1
  Demux9/1 -> Va/1(V)
  Vd/2(DVd_1) -> Mux1/3  "DVd_1"
  Gain/1 -> Switch5/1  "Equation (10)"
  V/1 -> Demux9/1
  Divide1/1 -> Mux2/2
  Mux2/1 -> Switch5/3  "Equation (11)"
  Constant/1 -> Mux2/1

== system Simulation/Motor Control and Resistance Estimation/Proposed method/R estimation/Low-pass filter ==
  Vpk : Inport
  BW : Inport  Port=2
  Product : Product
  Product1 : Product
  Sum1 : Sum  Inputs=+-  SaturateOnIntegerOverflow=on
  Sum2 : Sum  Inputs=+-  SaturateOnIntegerOverflow=on
  integrator : DiscreteIntegrator  gainval=1  SampleTime=-1  ICPrevOutput=DiscIntNeverNeededParam  ICPrevScaledInput=DiscIntNeverNeededParam
  integrator2 : DiscreteIntegrator  gainval=1  SampleTime=-1  ICPrevOutput=DiscIntNeverNeededParam  ICPrevScaledInput=DiscIntNeverNeededParam
  Out : Outport
  wires:
  integrator/1 -> Sum2/1, Sum1/2
  integrator2/1 -> Out/1, Sum2/2
  Product/1 -> integrator/1
  Sum1/1 -> Product/2
  Sum2/1 -> Product1/2
  Product1/1 -> integrator2/1
  BW/1 -> Product/1, Product1/1
  Vpk/1 -> Sum1/1

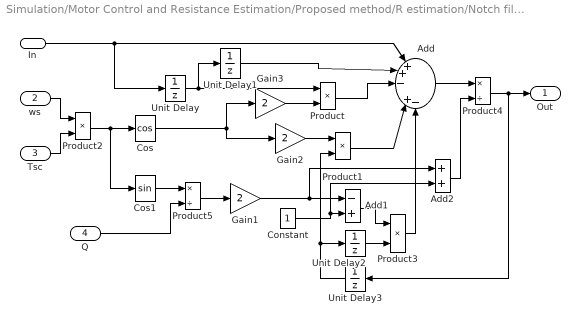
== system Simulation/Motor Control and Resistance Estimation/Proposed method/R estimation/Notch filter ==
  In : Inport
  ws : Inport  Port=2
  Tsc : Inport  Port=3
  Q : Inport  Port=4
  Add : Sum  Inputs=|++-|+-
  Add1 : Sum  Inputs=-+
  Add2 : Sum
  Constant : Constant
  Cos : Trigonometry  Operator=cos
  Cos1 : Trigonometry
  Gain1 : Gain  Gain=2
  Gain2 : Gain  Gain=2
  Gain3 : Gain  Gain=2
  Product{,1..3} (4 alike) : Product
  Product4 : Product  Inputs=*/
  Product5 : Product  Inputs=*/
  Unit Delay{,1..3} (4 alike) : UnitDelay  SampleTime=-1  HasFrameUpgradeWarning=on
  Out : Outport
  wires:
  Product4/1 -> Out/1, Unit Delay3/1
  Add2/1 -> Product4/2
  Add/1 -> Product4/1
  Cos1/1 -> Product5/1
  Gain3/1 -> Product/2
  Product/1 -> Add/3
  Product3/1 -> Add/5
  ws/1 -> Product2/1
  Constant/1 -> Add1/2, Add2/2
  Unit Delay2/1 -> Product3/2
  Cos/1 -> Gain2/1, Gain3/1
  Product1/1 -> Add/4
  Unit Delay/1 -> Product/1, Unit Delay1/1
  In/1 -> Unit Delay/1, Add/1
  Unit Delay3/1 -> Product1/2, Unit Delay2/1
  Unit Delay1/1 -> Add/2
  Product2/1 -> Cos/1, Cos1/1
  Product5/1 -> Gain1/1
  Add1/1 -> Product3/1
  Gain2/1 -> Product1/1
  Tsc/1 -> Product2/2
  Q/1 -> Product5/2
  Gain1/1 -> Add2/1, Add1/1

== system Simulation/Motor Control and Resistance Estimation/Proposed method/R estimation/Subsystem ==
  In : Inport
  Healthy_OPF : Inport  Port=2
  Demux : Demux  Outputs=[1 5]
  Mux2 : Mux  Inputs=2
  Switch : Switch  Criteria=u2 > Threshold  Threshold=0.5
  Out : Outport
  wires:
  Switch/1 -> Mux2/1
  In/1 -> Demux/1
  Demux/2 -> Mux2/2
  Healthy_OPF/1 -> Switch/2
  Demux/1 -> Switch/1
  Mux2/1 -> Out/1

== system Simulation/Motor Control and Resistance Estimation/Speed control loop/Subsystem2/Estimation of rotor-flux position and speed ==
  Id* : Inport
  Iq* : Inport  Port=2
  speed : Inport  Port=3
  Add5 : Sum
  Discrete-Time Integrator : DiscreteIntegrator  SampleTime=-1  ICPrevOutput=DiscIntNeverNeededParam  ICPrevScaledInput=DiscIntNeverNeededParam
  slip estimator : Subsystem
  theta_r : Outport  VectorParamsAs1DForOutWhenUnconnected=off
  "ws " : Outport  Port=2  VectorParamsAs1DForOutWhenUnconnected=off
  wires:
  Id*/1 -> slip estimator/2(Ids)
  slip estimator/1(slip speed) -> Add5/1
  Iq*/1 -> slip estimator/1(Iqs)
  speed/1 -> Add5/2
  Discrete-Time Integrator/1 -> theta_r/1
  Add5/1 -> "ws "/1, Discrete-Time Integrator/1

== system Simulation/Motor Control and Resistance Estimation/Speed control loop/Subsystem2/Inverse Park transformation ==
  "Id*, Iq*" : Inport
  "theta_r " : Inport  Port=2
  Cos : Trigonometry  Operator=cos
  "Inverse Park transform " : Subsystem
  Mux1 : Mux  Inputs=2
  Sin : Trigonometry
  "Ia*, Ib*" : Outport  VectorParamsAs1DForOutWhenUnconnected=off
  wires:
  "Id*, Iq*"/1 -> "Inverse Park transform "/1(dq)
  "Inverse Park transform "/1(ab) -> "Ia*, Ib*"/1
  "theta_r "/1 -> Cos/1, Sin/1
  Sin/1 -> Mux1/1
  Cos/1 -> Mux1/2
  Mux1/1 -> "Inverse Park transform "/2(sin_cos)

== system Simulation/Six-phase induction machine with extra per-phase stator resistances/Symmetrical six-phase induction machine with balanced stator resistances/Subsystem/a ==
  I : Inport
  Ip : powerlib/Electrical Sources/Controlled Current Source  Initialize=on  Source_Type=AC  Amplitude=0  Phase=0  Frequency=0  Measurements=None
  Rd : powerlib/Elements/Series RLC Branch  LConnTagsString=__new0  RConnTagsString=__new0  BranchType=R  Resistance=1e5  Inductance=1e-3  SetiL0=off  InitialCurrent=0  Capacitance=1e-6  Setx0=off  InitialVoltage=0  Measurements=None
  Vp : powerlib/Measurements/Voltage Measurement  PhasorSimulation=off  OutputType=Complex  PSBequivalent=0
  + : PMIOPort  Side=Left
  - : PMIOPort  Port=2  Side=Right
  V : Outport  VectorParamsAs1DForOutWhenUnconnected=off
  wires:
  Vp/1 -> V/1
  I/1 -> Ip/1
  connections:
  Vp/LConn2 -- Rd/RConn1 -- Ip/RConn1 -- -/RConn1
  Vp/LConn1 -- Rd/LConn1 -- Ip/LConn1 -- +/RConn1

== system Simulation/Six-phase induction machine with extra per-phase stator resistances/Symmetrical six-phase induction machine with balanced stator resistances/Subsystem/b ==
  I : Inport
  Ip : powerlib/Electrical Sources/Controlled Current Source  Initialize=on  Source_Type=AC  Amplitude=0  Phase=0  Frequency=0  Measurements=None
  Rd : powerlib/Elements/Series RLC Branch  LConnTagsString=__new0  RConnTagsString=__new0  BranchType=R  Resistance=1e5  Inductance=1e-3  SetiL0=off  InitialCurrent=0  Capacitance=1e-6  Setx0=off  InitialVoltage=0  Measurements=None
  Vp : powerlib/Measurements/Voltage Measurement  PhasorSimulation=off  OutputType=Complex  PSBequivalent=0
  + : PMIOPort  Side=Left
  - : PMIOPort  Port=2  Side=Right
  V : Outport  VectorParamsAs1DForOutWhenUnconnected=off
  wires:
  I/1 -> Ip/1
  Vp/1 -> V/1
  connections:
  Ip/LConn1 -- +/RConn1 -- Rd/LConn1 -- Vp/LConn1
  Rd/RConn1 -- Ip/RConn1 -- -/RConn1 -- Vp/LConn2

== system Simulation/Six-phase induction machine with extra per-phase stator resistances/Symmetrical six-phase induction machine with balanced stator resistances/Subsystem/c ==
  I : Inport
  Ip : powerlib/Electrical Sources/Controlled Current Source  Initialize=on  Source_Type=AC  Amplitude=0  Phase=0  Frequency=0  Measurements=None
  Rd : powerlib/Elements/Series RLC Branch  LConnTagsString=__new0  RConnTagsString=__new0  BranchType=R  Resistance=1e5  Inductance=1e-3  SetiL0=off  InitialCurrent=0  Capacitance=1e-6  Setx0=off  InitialVoltage=0  Measurements=None
  Vp : powerlib/Measurements/Voltage Measurement  PhasorSimulation=off  OutputType=Complex  PSBequivalent=0
  + : PMIOPort  Side=Left
  - : PMIOPort  Port=2  Side=Right
  V : Outport  VectorParamsAs1DForOutWhenUnconnected=off
  wires:
  Vp/1 -> V/1
  I/1 -> Ip/1
  connections:
  Vp/LConn2 -- Rd/RConn1 -- Ip/RConn1 -- -/RConn1
  Vp/LConn1 -- Rd/LConn1 -- +/RConn1 -- Ip/LConn1

== system Simulation/Six-phase induction machine with extra per-phase stator resistances/Symmetrical six-phase induction machine with balanced stator resistances/Subsystem/d ==
  I : Inport
  Ip : powerlib/Electrical Sources/Controlled Current Source  Initialize=on  Source_Type=AC  Amplitude=0  Phase=0  Frequency=0  Measurements=None
  Rd : powerlib/Elements/Series RLC Branch  LConnTagsString=__new0  RConnTagsString=__new0  BranchType=R  Resistance=1e5  Inductance=1e-3  SetiL0=off  InitialCurrent=0  Capacitance=1e-6  Setx0=off  InitialVoltage=0  Measurements=None
  Vp : powerlib/Measurements/Voltage Measurement  PhasorSimulation=off  OutputType=Complex  PSBequivalent=0
  + : PMIOPort  Side=Left
  - : PMIOPort  Port=2  Side=Right
  V : Outport  VectorParamsAs1DForOutWhenUnconnected=off
  wires:
  I/1 -> Ip/1
  Vp/1 -> V/1
  connections:
  +/RConn1 -- Ip/LConn1 -- Rd/LConn1 -- Vp/LConn1
  Ip/RConn1 -- Rd/RConn1 -- Vp/LConn2 -- -/RConn1

== system Simulation/Six-phase induction machine with extra per-phase stator resistances/Symmetrical six-phase induction machine with balanced stator resistances/Subsystem/e ==
  I : Inport
  Ip : powerlib/Electrical Sources/Controlled Current Source  Initialize=on  Source_Type=AC  Amplitude=0  Phase=0  Frequency=0  Measurements=None
  Rd : powerlib/Elements/Series RLC Branch  LConnTagsString=__new0  RConnTagsString=__new0  BranchType=R  Resistance=1e5  Inductance=1e-3  SetiL0=off  InitialCurrent=0  Capacitance=1e-6  Setx0=off  InitialVoltage=0  Measurements=None
  Vp : powerlib/Measurements/Voltage Measurement  PhasorSimulation=off  OutputType=Complex  PSBequivalent=0
  + : PMIOPort  Side=Left
  - : PMIOPort  Port=2  Side=Right
  V : Outport  VectorParamsAs1DForOutWhenUnconnected=off
  wires:
  Vp/1 -> V/1
  I/1 -> Ip/1
  connections:
  Vp/LConn2 -- Rd/RConn1 -- Ip/RConn1 -- -/RConn1
  Vp/LConn1 -- Rd/LConn1 -- Ip/LConn1 -- +/RConn1

== system Simulation/Six-phase induction machine with extra per-phase stator resistances/Symmetrical six-phase induction machine with balanced stator resistances/Subsystem/f ==
  I : Inport
  Ip : powerlib/Electrical Sources/Controlled Current Source  Initialize=on  Source_Type=AC  Amplitude=0  Phase=0  Frequency=0  Measurements=None
  Rd : powerlib/Elements/Series RLC Branch  LConnTagsString=__new0  RConnTagsString=__new0  BranchType=R  Resistance=1e5  Inductance=1e-3  SetiL0=off  InitialCurrent=0  Capacitance=1e-6  Setx0=off  InitialVoltage=0  Measurements=None
  Vp : powerlib/Measurements/Voltage Measurement  PhasorSimulation=off  OutputType=Complex  PSBequivalent=0
  + : PMIOPort  Side=Left
  - : PMIOPort  Port=2  Side=Right
  V : Outport  VectorParamsAs1DForOutWhenUnconnected=off
  wires:
  I/1 -> Ip/1
  Vp/1 -> V/1
  connections:
  +/RConn1 -- Ip/LConn1 -- Rd/LConn1 -- Vp/LConn1
  Ip/RConn1 -- Rd/RConn1 -- Vp/LConn2 -- -/RConn1

== system Simulation/Motor Control and Resistance Estimation/Proposed method/Generation of time sequence for injection/Time delay 1/Detect rising edge ==
  In : Inport
  Compare To Constant : simulink/Logic and Bit Operations/Compare To Constant  relop=>=  const=1  OutDataTypeStr=boolean
  Compare To Constant1 : simulink/Logic and Bit Operations/Compare To Constant  relop=<  const=1  OutDataTypeStr=boolean
  Logical Operator : Logic  AllPortsSameDT=off  OutDataTypeStr=boolean
  delay : UnitDelay  SampleTime=-1
  Out : Outport
  wires:
  delay/1 -> Compare To Constant1/1
  Logical Operator/1 -> Out/1
  In/1 -> Compare To Constant/1, delay/1
  Compare To Constant/1 -> Logical Operator/1
  Compare To Constant1/1 -> Logical Operator/2

== system Simulation/Motor Control and Resistance Estimation/Proposed method/Generation of time sequence for injection/Time delay 2/Detect rising edge ==
  In : Inport
  Compare To Constant : simulink/Logic and Bit Operations/Compare To Constant  relop=>=  const=1  OutDataTypeStr=boolean
  Compare To Constant1 : simulink/Logic and Bit Operations/Compare To Constant  relop=<  const=1  OutDataTypeStr=boolean
  Logical Operator : Logic  AllPortsSameDT=off  OutDataTypeStr=boolean
  delay : UnitDelay  SampleTime=-1
  Out : Outport
  wires:
  Compare To Constant1/1 -> Logical Operator/2
  Compare To Constant/1 -> Logical Operator/1
  In/1 -> delay/1, Compare To Constant/1
  Logical Operator/1 -> Out/1
  delay/1 -> Compare To Constant1/1
